simulink subsystem "PowerGain"  (R2025a)
settings: Solver=VariableStepAuto  StartTime=0.0  StopTime=10.0  RelTol=1e-3
model mask{gain=0}
settings Model: Creator=Глеб  LastModifiedBy=Глеб

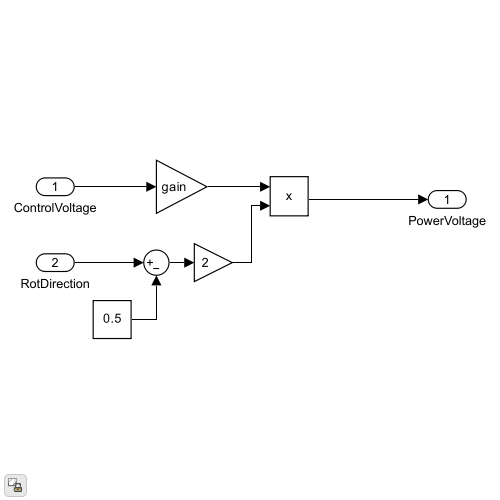
[thumbnail: Simulink's stored preview of the top-level diagram]
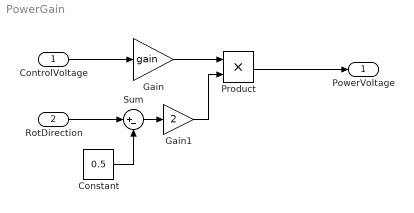
== system PowerGain ==
  ControlVoltage : Inport
  RotDirection : Inport  Port=2  OutDataTypeStr=boolean
  Constant : Constant  Value=0.5
  Gain : Gain  Gain=gain
  Gain1 : Gain  Gain=2
  Product : Product
  Sum : Sum  Inputs=|+-
  PowerVoltage : Outport
  wires:
  ControlVoltage/1 -> Gain/1
  Gain/1 -> Product/1
  Product/1 -> PowerVoltage/1
  RotDirection/1 -> Sum/1
  Constant/1 -> Sum/2
  Sum/1 -> Gain1/1
  Gain1/1 -> Product/2
